simulink library "Custom_Valve_Choices_Lib"  (R2013a)
settings: Solver=ode45  SolverMode=SingleTasking  StartTime=0.0  StopTime=10.0  RelTol=1e-3
libraries: fl_lib x57, sh_lib x10, nesl_utility x8, Custom_Valve_Orifices_Lib x3, Custom_Valve_Choices_Lib x1
(part 2 of 2)

== system Custom_Valve_Choices_Lib/Servovalve Center/Valve/Orifices ==
  No Force : Custom_Valve_Orifices_Lib/No Force  or_width=orifice_width  x0_PA=x0_orifice_PA  x0_PB=x0_orifice_PB  x0_AT=x0_orifice_AT  x0_BT=x0_orifice_BT
  P : PMIOPort  Port=1  Side=Left
  T : PMIOPort  Port=2  Side=Left
  A : PMIOPort  Port=3  Side=Right
  Spool : PMIOPort  Port=4  Side=Right
  B : PMIOPort  Port=5  Side=Right
  connections:
  No Force/LConn1 -- P/RConn1
  No Force/LConn2 -- T/RConn1
  No Force/RConn1 -- A/RConn1
  No Force/RConn2 -- Spool/RConn1
  No Force/RConn3 -- B/RConn1

== system Custom_Valve_Choices_Lib/Servovalve Center/Valve/P_Cyl_B1 ==
  Ideal Translational Motion Sensor : fl_lib/Mechanical/Mechanical Sensors/Ideal Translational Motion Sensor  Tag=Factory Generic  offset=0 m  v_Log=off  f_Log=off  x_Log=off  LocalVarNames=|v|f|x  LocalVarDescs=|v|f|x  LocalVarLogging=[]
  MTR3 : fl_lib/Mechanical/Translational Elements/Mechanical Translational Reference  Tag=Factory Generic  f_Log=off  LocalVarNames=|f  LocalVarDescs=|f  LocalVarLogging=[]
  PS-Simulink Converter2 : nesl_utility/PS-Simulink Converter  PhysicalDomain=network_engine_domain  LeftPortType=input  RightPortType=output  SubClassName=ps_output  PseudoPeriodic=off  Frequencies=[]  Unit=mm  AffineConversion=off
  X : PMIOPort  Port=1  Side=Left
  tag scope: Spool_x=global
  wires:
  PS-Simulink Converter2/1 -> [Spool_x]  "Spool_Position"
  connections:
  Ideal Translational Motion Sensor/RConn3 -- PS-Simulink Converter2/LConn1
  X/RConn1 -- Ideal Translational Motion Sensor/LConn1
  MTR3/LConn1 -- Ideal Translational Motion Sensor/RConn1

== system Custom_Valve_Choices_Lib/Servovalve Flapper/Diagram/Diagram ==

== system Custom_Valve_Choices_Lib/Servovalve Flapper/Valve/Orifices ==
  With Force : Custom_Valve_Orifices_Lib/With Force  or_width=orifice_width  x0_PA=x0_orifice_PA  x0_PB=x0_orifice_PB  x0_AT=x0_orifice_AT  x0_BT=x0_orifice_BT  rad_clearance=spool_rad_clear
  P : PMIOPort  Port=1  Side=Left
  T : PMIOPort  Port=2  Side=Left
  A : PMIOPort  Port=3  Side=Right
  Spool : PMIOPort  Port=4  Side=Right
  B : PMIOPort  Port=5  Side=Right
  connections:
  With Force/LConn1 -- P/RConn1
  With Force/LConn2 -- T/RConn1
  With Force/RConn1 -- A/RConn1
  With Force/RConn2 -- Spool/RConn1
  With Force/RConn3 -- B/RConn1

== system Custom_Valve_Choices_Lib/Servovalve Flapper/Valve/P_Cyl_B2 ==
  Ideal Translational Motion Sensor : fl_lib/Mechanical/Mechanical Sensors/Ideal Translational Motion Sensor  Tag=Factory Generic  offset=0 m  v_Log=off  f_Log=off  x_Log=off  LocalVarNames=|v|f|x  LocalVarDescs=|v|f|x  LocalVarLogging=[]
  MTR3 : fl_lib/Mechanical/Translational Elements/Mechanical Translational Reference  Tag=Factory Generic  f_Log=off  LocalVarNames=|f  LocalVarDescs=|f  LocalVarLogging=[]
  PS-Simulink Converter2 : nesl_utility/PS-Simulink Converter  PhysicalDomain=network_engine_domain  LeftPortType=input  RightPortType=output  SubClassName=ps_output  PseudoPeriodic=off  Frequencies=[]  Unit=mm  AffineConversion=off
  X : PMIOPort  Port=1  Side=Left
  tag scope: Spool_x=global
  wires:
  PS-Simulink Converter2/1 -> [Spool_x]  "Spool_Position"
  connections:
  Ideal Translational Motion Sensor/RConn3 -- PS-Simulink Converter2/LConn1
  X/RConn1 -- Ideal Translational Motion Sensor/LConn1
  MTR3/LConn1 -- Ideal Translational Motion Sensor/RConn1
